simulink model "Posture_Regulation_Singularity"  (R2022b)
settings: Solver=FixedStepAuto  StartTime=0.0  StopTime=10.0  MaxStep=0.1  RelTol=1e-3
undefined symbols (not defined in the file): K, theta_f, theta_i, x_f, x_i, y_f, y_i
libraries: simulink_extras x2
settings Model: Creator=Musta  LastModifiedBy=Musta

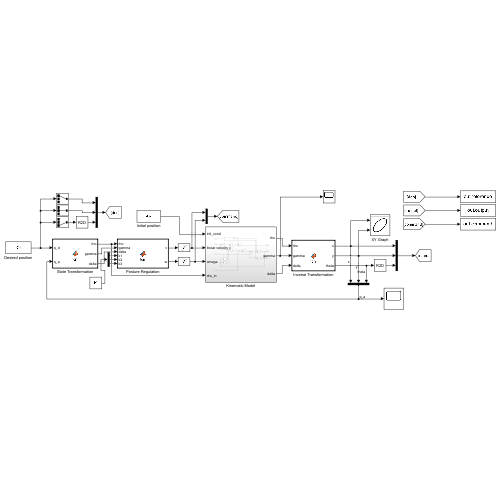
[thumbnail: Simulink's stored preview of the top-level diagram]
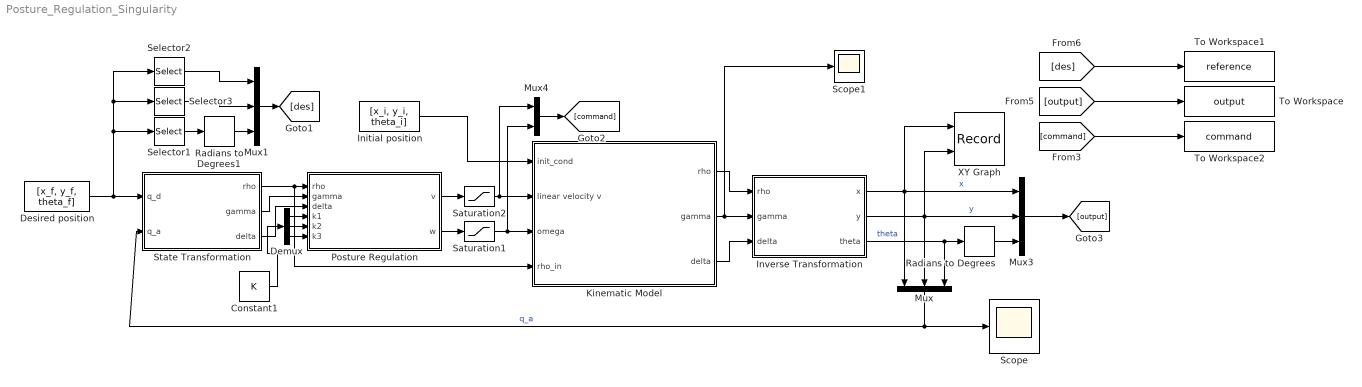
== system Posture_Regulation_Singularity ==
  Constant1 : Constant  Value=K
  Demux : Demux  Outputs=3
  Desired position : Constant  Value=[x_f, y_f, theta_f]
  Initial position : Constant  Value=[x_i, y_i, theta_i]
  Inverse Transformation : MATLAB Function  TreatAsAtomicUnit=on
  Kinematic Model : Subsystem
  Mux : Mux  Inputs=3
  Mux1 : Mux  Inputs=3
  Mux3 : Mux  Inputs=3
  Mux4 : Mux  Inputs=2
  Posture Regulation : MATLAB Function  TreatAsAtomicUnit=on
  Radians to Degrees : simulink_extras/Transformations/Radians to Degrees
  Radians to Degrees1 : simulink_extras/Transformations/Radians to Degrees
  Saturation1 : Saturate  UpperLimit=2  LowerLimit=-2
  Saturation2 : Saturate  UpperLimit=2  LowerLimit=-2
  Scope : Scope
  Scope1 : Scope
  Selector1 : Selector  InputPortWidth=3  IndexOptions=Index vector (dialog)  Indices=3  OutputSizes=1
  Selector2 : Selector  InputPortWidth=3  IndexOptions=Index vector (dialog)  Indices=1  OutputSizes=1
  Selector3 : Selector  InputPortWidth=3  IndexOptions=Index vector (dialog)  Indices=2  OutputSizes=1
  State Transformation : MATLAB Function  TreatAsAtomicUnit=on
  To Workspace : ToWorkspace  VariableName=output  SaveFormat=Structure With Time  SampleTime=-1
  To Workspace1 : ToWorkspace  VariableName=reference  SaveFormat=Structure With Time  SampleTime=-1
  To Workspace2 : ToWorkspace  VariableName=command  SaveFormat=Structure With Time  SampleTime=-1
  XY Graph : Record  FileSettingsInternal="{\"entries\":[{\"content\":{\"excelSettings\":{\"content\":{},\"type\":\"Streamout.ExcelSettings\"}},\"type\":\"Streamout.FileSettingStorage\",\"uuid\":\"c67a5f3d-077a-4888-809e-c2fef9ca71b1\"}],\"packageUris\":[\"http://schema.mathworks.com/mf0/streamout_blocks/R2020a\"],\"version\":\"1.0\"}"  Layout=[1 1]  SignalsInternal="{\"entries\":[{\"content\":{\"signals\":[{\"content\":{\"blockPath\":[\"Posture_Regulation_Singularity/XY Graph\"],\"channel\":[],\"dimensions\":[1],\"domain\":\"Posture_Regulation_Singularity/XY Graph\",\"lineColor\":\"#a2142f\",\"plots\":[1],\"port\":1,\"sid\":[\"\"],\"signalID\":305,\"signalName\":\"x\"},\"type\":\"RecordBlkView.Signal\",\"uuid\":\"d76dd3e0-b632-4dfe-a97e-b48e5c8288c6\"},{\"content\":{\"blockPath\":[\"Posture_Regulation_Singularity/XY Graph\"],\"channel\":[],\"dimensions\":[1],\"domain\":\"Posture_Regulation_Singularity/XY Graph\",\"lineColor\":\"#139fff\",\"plots\":[1],\"port\":2,\"sid\":[\"\"],\"signalID\":309,\"signalName\":\"y\"},\"type\":\"RecordBlkView.Signal\",\"uuid\":\"ed3713af-a470-46c0-aeb4-658ab6e5792c\"}]},\"type\":\"RecordBlkView.InputSignals\",\"uuid\":\"3a0e6c79-f3e4-4922-8768-8ca172808b3a\"}],\"packageUris\":[\"http://schema.mathworks.com/mf0/streamout_blocks/R2020a\"],\"version\":\"1.0\"}"  VisualizationBindings="{\"xyplotplugin\":{\"info\":[{\"series\":[{\"bindingParametersList\":[{\"parameter\":\"X-Axis\",\"signalID\":305,\"signalName\":\"x\"},{\"parameter\":\"Y-Axis\",\"signalID\":309,\"signalName\":\"y\"}],\"seriesID\":1406}],\"subplotID\":1}]}}"  CompatibilityTag=XY
  wires:
  Selector2/1 -> Mux1/1
  [output] -> To Workspace/1
  Selector1/1 -> Radians to Degrees1/1
  [command] -> To Workspace2/1
  Inverse Transformation/2(y) -> Mux3/2, Mux/2, XY Graph/2  "y"
  Selector3/1 -> Mux1/2
  Kinematic Model/2(gamma) -> Scope1/1, Inverse Transformation/2(gamma)
  Posture Regulation/2(w) -> Saturation1/1
  Radians to Degrees1/1 -> Mux1/3
  Kinematic Model/1(rho) -> Inverse Transformation/1(rho)
  Inverse Transformation/1(x) -> Mux/1, Mux3/1, XY Graph/1  "x"
  [des] -> To Workspace1/1
  Saturation2/1 -> Mux4/1, Kinematic Model/2(linear velocity v)
  State Transformation/3(delta) -> Posture Regulation/3(delta)
  State Transformation/1(rho) -> Posture Regulation/1(rho), Kinematic Model/4(rho_in)
  Desired position/1 -> Selector2/1, Selector3/1, Selector1/1, State Transformation/1(q_d)
  Mux1/1 -> [des]
  State Transformation/2(gamma) -> Posture Regulation/2(gamma)
  Mux/1 -> Scope/1, State Transformation/2(q_a)  "q_a"
  Initial position/1 -> Kinematic Model/1(init_cond)
  Kinematic Model/3(delta) -> Inverse Transformation/3(delta)
  Saturation1/1 -> Mux4/2, Kinematic Model/3(omega)
  Mux4/1 -> [command]
  Inverse Transformation/3(theta) -> Mux/3, Radians to Degrees/1  "theta"
  Posture Regulation/1(v) -> Saturation2/1
  Radians to Degrees/1 -> Mux3/3
  Mux3/1 -> [output]
  Demux/1 -> Posture Regulation/4(k1)
  Demux/2 -> Posture Regulation/5(k2)
  Demux/3 -> Posture Regulation/6(k3)
  Constant1/1 -> Demux/1

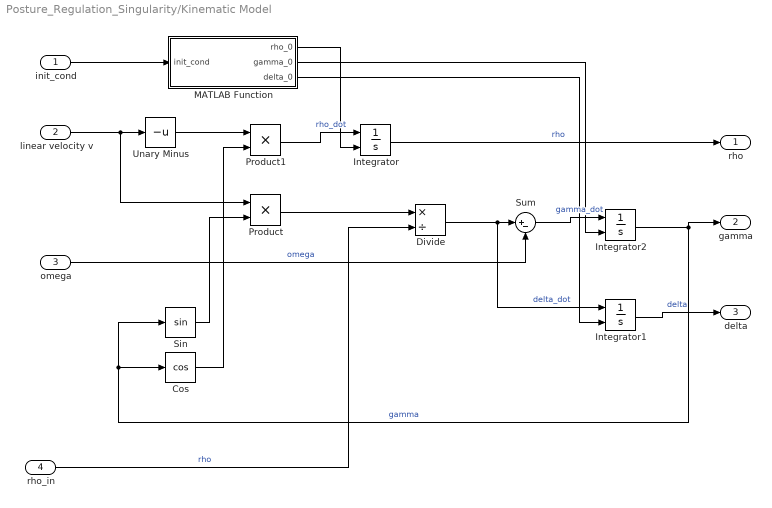
== system Posture_Regulation_Singularity/Kinematic Model ==
  init_cond : Inport
  linear velocity v : Inport  Port=2
  omega : Inport  Port=3
  rho_in : Inport  Port=4
  Cos : Trigonometry  Operator=cos
  Divide : Product  Inputs=*/
  Integrator : Integrator  InitialConditionSource=external
  Integrator1 : Integrator  InitialConditionSource=external
  Integrator2 : Integrator  InitialConditionSource=external
  MATLAB Function : MATLAB Function  TreatAsAtomicUnit=on
  Product : Product
  Product1 : Product
  Sin : Trigonometry
  Sum : Sum  Inputs=|+-
  Unary Minus : UnaryMinus
  rho : Outport
  gamma : Outport  Port=2
  delta : Outport  Port=3
  wires:
  Sum/1 -> Integrator2/1  "gamma_dot"
  Cos/1 -> Product1/2
  Unary Minus/1 -> Product1/1
  linear velocity v/1 -> Product/1, Unary Minus/1
  Product1/1 -> Integrator/1  "rho_dot"
  Integrator/1 -> rho/1  "rho"
  Sin/1 -> Product/2
  Product/1 -> Divide/1
  Divide/1 -> Integrator1/1, Sum/1  "delta_dot"
  omega/1 -> Sum/2  "omega"
  Integrator2/1 -> gamma/1, Cos/1, Sin/1  "gamma"
  Integrator1/1 -> delta/1  "delta"
  rho_in/1 -> Divide/2  "rho"
  init_cond/1 -> MATLAB Function/1(init_cond)
  MATLAB Function/1(rho_0) -> Integrator/2
  MATLAB Function/2(gamma_0) -> Integrator2/2
  MATLAB Function/3(delta_0) -> Integrator1/2

== matlab function Posture_Regulation_Singularity/Inverse Transformation ==
  data: x output; rho input; y output; gamma input; delta input; theta output
function [x,y,theta] = fcn(rho,gamma,delta)

    x = - rho * cos(delta);
    y = - rho * sin(delta);
    theta = delta - gamma;
    
end

== matlab function Posture_Regulation_Singularity/State Transformation ==
  data: q_d input; rho output; q_a input; gamma output; delta output
function [rho,gamma,delta] = fcn(q_d, q_a)

    e_x = q_d(1) - q_a(1);
    e_y = q_d(2) - q_a(2);
    e_theta = q_d(3) - q_a(3);
   
    rho = sqrt(e_x^2 + e_y^2);
    gamma = mod(atan2(e_y,e_x),2*pi) - q_a(3);
    delta = gamma - e_theta;

end

== matlab function Posture_Regulation_Singularity/Posture Regulation ==
  data: v output; w output; rho input; gamma input; delta input; k1 input; k2 input; k3 input
function [v,w] = fcn(rho,gamma,delta,k1,k2,k3)

    v = k1 * rho * cos(gamma);
    w = k2 * gamma + k1 *(sin(gamma)*cos(gamma))*(gamma + k3 * delta)/gamma;

    % handling the singularity of v 
    if abs(v) < 10^-4
        if v > 0
            v = 10^-4;
        else
            v = -10^-4;
        end   
    end    

end

== matlab function Posture_Regulation_Singularity/Kinematic Model/MATLAB Function ==
  data: init_cond input; rho_0 output; gamma_0 output; delta_0 output
function [rho_0, gamma_0, delta_0] = fcn(init_cond)

x_0 = init_cond(1);
y_0 = init_cond(2);
theta_0 = init_cond(3);


rho_0 = sqrt(x_0^2 + y_0^2);
gamma_0 = atan2(y_0,x_0) - theta_0 + pi;
delta_0 = gamma_0 + theta_0;
